simulink model "full_state"  (R2025a)
settings: Solver=VariableStepAuto  StartTime=0.0  StopTime=15  RelTol=1e-3
values from neighbouring files (symbols this model uses):
  A_real = double(A_real)    [Controls_proj.m]
  B_real = double(B_real)    [Controls_proj.m]
  C_sens = [1 0 0 0 0 0 ; 0 0 1 0 0 0]    [Controls_proj.m]
  K = lqr(A_real,B_real,Q,R_lqr)    [Controls_proj.m]
  Ke = place(A_real',C_sens',observer_poles)'    [Controls_proj.m]
settings Model: Creator=retqrd  LastModifiedBy=retqrd

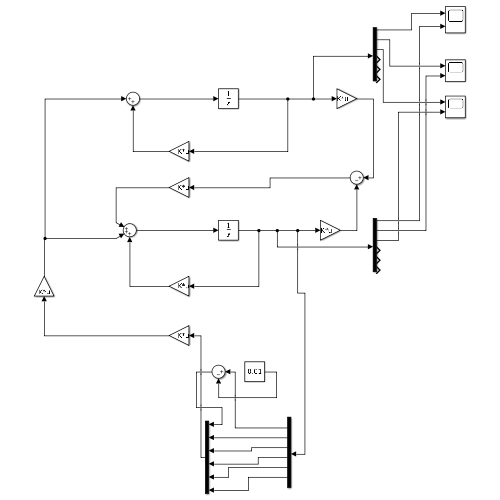
[thumbnail: Simulink's stored preview of the top-level diagram]
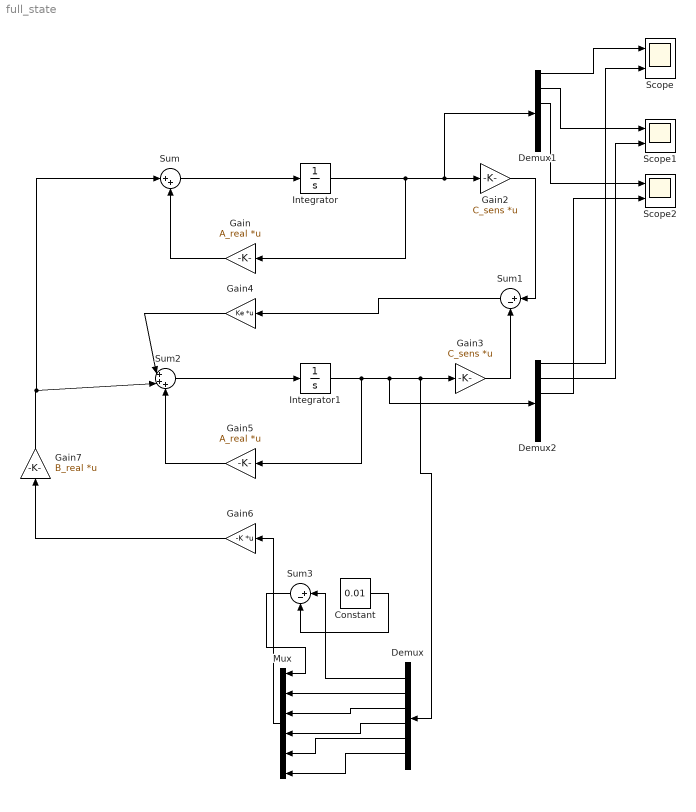
== system full_state ==
  Constant : Constant  Value=0.01
  Demux : Demux  Outputs=6
  Demux1 : Demux  Outputs=6
  Demux2 : Demux  Outputs=6
  Gain : Gain  Gain=A_real  Multiplication=Matrix(K*u)
  Gain2 : Gain  Gain=C_sens  Multiplication=Matrix(K*u)
  Gain3 : Gain  Gain=C_sens  Multiplication=Matrix(K*u)
  Gain4 : Gain  Gain=Ke  Multiplication=Matrix(K*u)
  Gain5 : Gain  Gain=A_real  Multiplication=Matrix(K*u)
  Gain6 : Gain  Gain=-K  Multiplication=Matrix(K*u)
  Gain7 : Gain  Gain=B_real  Multiplication=Matrix(K*u)
  Integrator : Integrator  InitialCondition=[0;0;4*pi/180;0;0;0];
  Integrator1 : Integrator  InitialCondition=[0;0;pi/180;0;0;0];
  Mux : Mux  Inputs=6
  Scope : Scope  NumInputPorts=2
      settings: ActiveDisplayYMinimum=-0.075417018476501479  ActiveDisplayYMaximum=0.068206793798433973
  Scope1 : Scope  NumInputPorts=2
      settings: ActiveDisplayYMinimum=0.23085704540244195  ActiveDisplayYMaximum=1.0826969513748308
  Scope2 : Scope  NumInputPorts=2
      settings: ActiveDisplayYMinimum=-0.025283783657004927  ActiveDisplayYMaximum=0.099158365022268713  DataLoggingVariableName=ScopeData2
  Sum : Sum  Inputs=|++
  Sum1 : Sum  Inputs=|+-
  Sum2 : Sum  Inputs=|+++
  Sum3 : Sum  Inputs=|+-
  wires:
  Integrator/1 -> Demux1/1, Gain2/1, Gain/1
  Sum/1 -> Integrator/1
  Gain/1 -> Sum/2
  Gain2/1 -> Sum1/1
  Gain3/1 -> Sum1/2
  Sum2/1 -> Integrator1/1
  Integrator1/1 -> Gain5/1, Demux2/1, Demux/1, Gain3/1
  Sum1/1 -> Gain4/1
  Gain4/1 -> Sum2/1
  Gain5/1 -> Sum2/3
  Gain6/1 -> Gain7/1
  Gain7/1 -> Sum/1, Sum2/2
  Demux/6 -> Mux/6
  Demux/5 -> Mux/5
  Demux/4 -> Mux/4
  Demux/3 -> Mux/3
  Demux/2 -> Mux/2
  Demux/1 -> Sum3/1
  Constant/1 -> Sum3/2
  Sum3/1 -> Mux/1
  Mux/1 -> Gain6/1
  Demux1/1 -> Scope/1
  Demux1/2 -> Scope1/1
  Demux1/3 -> Scope2/1
  Demux2/1 -> Scope/2
  Demux2/2 -> Scope1/2
  Demux2/3 -> Scope2/2
